simulink model "simulation"  (R2022b)
settings: Solver=VariableStepAuto  StartTime=0.0  StopTime=2000  RelTol=1e-3
undefined symbols (not defined in the file): AeroDragCoeff, airDensity, frontArea, gravity, inclineAngle, magnitude, massVeh, rollingResistCoeff
libraries: autolibshared x1, Driver_Glider_Library x1, slpidlib x1
settings Model: Creator=alexa  LastModifiedBy=alexa

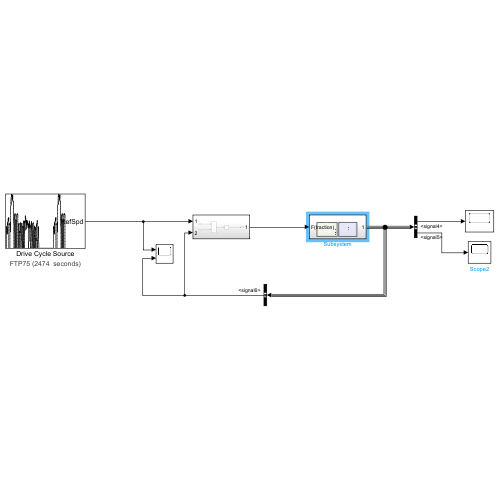
[thumbnail: Simulink's stored preview of the top-level diagram]
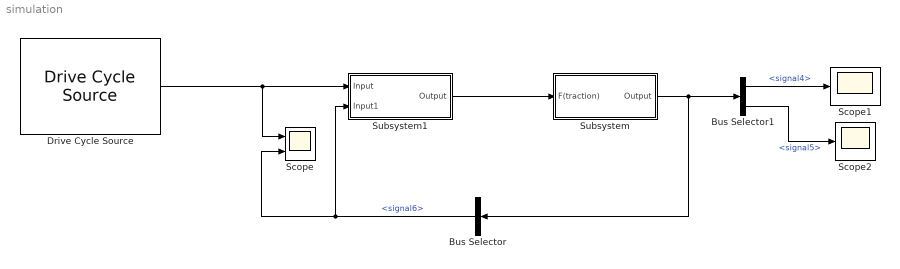
== system simulation ==
  Bus Selector : BusSelector  OutputSignals=signal6
  Bus Selector1 : BusSelector  OutputSignals=signal4,signal5
  Drive Cycle Source : autolibshared/Drive Cycle Source  cycleVar=FTP75  fileVar=cycleFTP75.mat  tfinal="2474  seconds"  cycleRepeat=off  outAccPort=off  outGearPort=off  gearList=No gear data  t_wot1=5  xdot_woto=0  xdot_wot1=30  t_wot2=20  xdot_wot2=0  t_wotend=30  srcUnit=m/s  outUnit=m/s  srcAccUnit=m/s/s  outAccUnit=m/s^2  dt=0  aMode=1  faultOption=off  velBnd=2  velBndUnit=mph  inUnit=m/s  timeBnd=1  failOption=off  stopSim=off  maxFaultCnt=10  maxFaultTime=2  maxTotFaultTime=15  traceOption=off  dtTrace=1  traceWindow=10  lastDCname=Heavy Heavy-Duty Diesel Truck (HHDDT) - Cruise Mode  lastOutUnit=mph  lastDT=2000  lastTB=1  lastSB=2  forceCalcBound=off
  Scope : Scope  NumInputPorts=2
  Scope1 : Scope
  Scope2 : Scope
  Subsystem : Subsystem
  Subsystem1 : Subsystem
  wires:
  Drive Cycle Source/1 -> Scope/1, Subsystem1/1(Input)
  Bus Selector/1 -> Scope/2, Subsystem1/2(Input1)  "<signal6>"
  Subsystem1/1(Output) -> Subsystem/1(F(traction))
  Subsystem/1(Output) -> Bus Selector1/1, Bus Selector/1
  Bus Selector1/1 -> Scope1/1  "<signal4>"
  Bus Selector1/2 -> Scope2/1  "<signal5>"

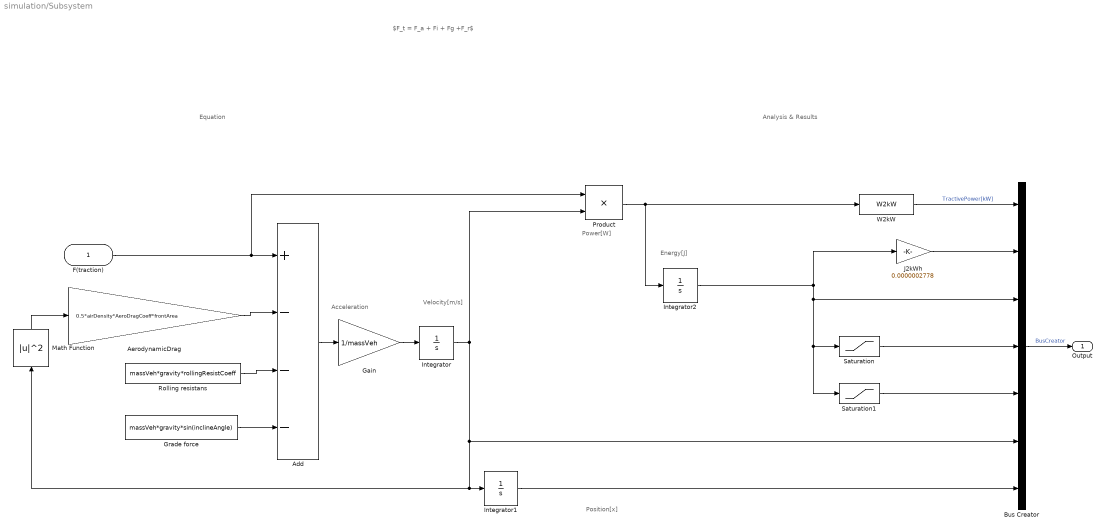
== system simulation/Subsystem ==
  note: Analysis & Results
  note: Power[W]
  note: Equation
  note: Velocity[m/s]
  note: Energy[J]
  note: Position[x]
  note: $F_t = F_a + Fi + Fg +F_r$
  note: Acceleration
  F(traction) : Inport
  Add : Sum  Inputs=+---
  AerodynamicDrag : Gain  Gain=0.5*airDensity*AeroDragCoeff*frontArea
  Bus Creator : BusCreator  Inputs=7
  Gain : Gain  Gain=1/massVeh
  Grade force : Constant  Value=massVeh*gravity*sin(inclineAngle)
  Integrator : Integrator
  Integrator1 : Integrator
  Integrator2 : Integrator
  J2kWh : Gain  Gain=0.0000002778
  Math Function : Math  Operator=magnitude^2
  Product : Product
  Rolling resistans : Constant  Value=massVeh*gravity*rollingResistCoeff
  Saturation : Saturate  UpperLimit=inf  LowerLimit=0
  Saturation1 : Saturate  UpperLimit=0  LowerLimit=-inf
  W2kW : Driver_Glider_Library/Glider/W2kW  SystemSampleTime=-1  VariantActivationTime=update diagram  Latency=0  AutoFrameSizeCalculation=off
  Output : Outport
  wires:
  Product/1 -> W2kW/1, Integrator2/1
  Add/1 -> Gain/1
  AerodynamicDrag/1 -> Add/2
  Gain/1 -> Integrator/1
  Math Function/1 -> AerodynamicDrag/1
  F(traction)/1 -> Product/1, Add/1
  Integrator/1 -> Bus Creator/6, Integrator1/1, Math Function/1, Product/2
  Saturation/1 -> Bus Creator/4
  Integrator1/1 -> Bus Creator/7
  Grade force/1 -> Add/4
  Saturation1/1 -> Bus Creator/5
  Rolling resistans/1 -> Add/3
  Integrator2/1 -> J2kWh/1, Saturation1/1, Saturation/1, Bus Creator/3
  J2kWh/1 -> Bus Creator/2
  Bus Creator/1 -> Output/1  "BusCreator"
  W2kW/1 -> Bus Creator/1  "TractivePower[kW]"

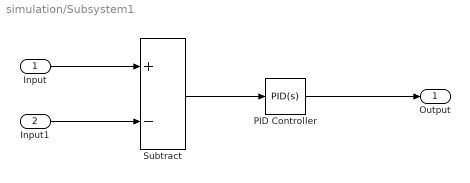
== system simulation/Subsystem1 ==
  Input : Inport
  Input1 : Inport  Port=2
  PID Controller : slpidlib/PID Controller  Controller=PID  Form=Parallel  TimeDomain=Continuous-time  UseExternalTs=off  SampleTime=-1  IntegratorMethod=Forward Euler  FilterMethod=Forward Euler  ControllerParametersSource=internal  P=7500  I=1  UseKiTs=off  D=0  N=100  UseFilter=on  TunerSelectOption=Transfer Function Based (PID Tuner App)  InitialConditionSource=internal  InitialConditionForIntegrator=0  InitialConditionForFilter=0  DifferentiatorICPrevScaledInput=0  ExternalReset=none  TrackingMode=off  Kt=1  LimitOutput=off  SatLimitsSource=internal  UpperSaturationLimit=inf  LowerSaturationLimit=-inf  LinearizeAsGain=on  AntiWindupMode=none  Kb=1  LimitIntegrator=off  UpperIntegratorSaturationLimit=inf  LowerIntegratorSaturationLimit=-inf  POutMin=[]  POutMax=[]  IOutMin=[]  IOutMax=[]  DOutMin=[]  DOutMax=[]  NOutMin=[]  NOutMax=[]  SumOutMin=[]  SumOutMax=[]  SaturationOutMin=[]  SaturationOutMax=[]  PParamMin=[]  PParamMax=[]  IParamMin=[]  IParamMax=[]  DParamMin=[]  DParamMax=[]  NParamMin=[]  NParamMax=[]  KbParamMin=[]  KbParamMax=[]  KtParamMin=[]  KtParamMax=[]  KbOutMin=[]  KbOutMax=[]  KtOutMin=[]  KtOutMax=[]  IntegratorOutMin=[]  IntegratorOutMax=[]  FilterOutMin=[]  FilterOutMax=[]  SumI1OutMin=[]  SumI1OutMax=[]  SumI2OutMin=[]  SumI2OutMax=[]  SumI3OutMin=[]  SumI3OutMax=[]  SumI4OutMin=[]  SumI4OutMax=[]  SumDOutMin=[]  SumDOutMax=[]  DifferentiatorOutMin=[]  DifferentiatorOutMax=[]  FilterDiffOutCoefMin=[]  FilterDiffOutCoefMax=[]  ReciprocalOutMin=[]  ReciprocalOutMax=[]  SumDenOutMin=[]  SumDenOutMax=[]  SumNumOutMin=[]  SumNumOutMax=[]  DivideOutMin=[]  DivideOutMax=[]  UdiffTsProdOutMin=[]  UdiffTsProdOutMax=[]  NTsProdOutMin=[]  NTsProdOutMax=[]  UintegralTsProdOutMin=[]  UintegralTsProdOutMax=[]  UngainTsProdOutMin=[]  UngainTsProdOutMax=[]  ClampingZeroOutDataTypeStr=Inherit: Inherit via back propagation  ClampingZeroOutMin=[]  ClampingZeroOutMax=[]  FilterDenConstantOutDataTypeStr=Inherit: Inherit via back propagation  FilterDenConstantOutMin=[]  FilterDenConstantOutMax=[]  PCopyOutDataTypeStr=Inherit: Inherit via back propagation  PCopyOutMin=[]  PCopyOutMax=[]  NCopyOutDataTypeStr=Inherit: Inherit via back propagation  NCopyOutMin=[]  NCopyOutMax=[]  IntegratorContinuousStateAttributes=''  IntegratorStateMustResolveToSignalObject=off  IntegratorRTWStateStorageClass=Auto  FilterContinuousStateAttributes=''  FilterStateMustResolveToSignalObject=off  FilterRTWStateStorageClass=Auto  ParallelPVariant=InternalParameters  IdealPVariant=Disabled  IVariant=InternalParameters  DVariant=InternalParameters  IntegratorVariant=Continuous  SatVariant=Disabled  AWVariant=Passthrough  PCopyVariant=Disabled  TRVariant=Disabled  FdbkBlocksVariant=Forward  IdealPFdbkVariant=Disabled  SatFdbkVariant=Disabled  DerivativeFilterVariant=ContFilter  NVariant=InternalParameters  NCopyVariant=Disabled  FilterICVariant=InternalICsFilter  IntegratorICVariant=InternalICs  ExternalResetVariant=Disabled  TRSumVariant=Passthrough  SumFdbkVariant=Disabled  SumVariant=Sum_PID  TsampFilterVariant=InternalTs  TsampNgainVariant=Passthrough  TsampIntegralVariant=Passthrough  ExternalSaturationOutDataTypeStr=Inherit: Same as second input
  Subtract : Sum  Inputs=+-
  Output : Outport
  wires:
  Input/1 -> Subtract/1
  PID Controller/1 -> Output/1
  Input1/1 -> Subtract/2
  Subtract/1 -> PID Controller/1
